simulink model "Solar_App"  (R2020a)
settings: Solver=VariableStepAuto  StartTime=0.0  StopTime=10.0  RelTol=1e-3
libraries: ee_lib x81, powerlib x29, fl_lib x4, nesl_utility x3, powerlib_extras x1
settings Model: Creator=momit  LastModifiedBy=royde
settings DataIOCC: ReturnWorkspaceOutputs=off
settings DebuggingCC: ArithmeticOperatorsInVariantConditions=warning
settings SFSimCC: SimUseLocalCustomCode=off  CustomCodeUndefinedFunction=UseInterfaceOnly
settings RTWCC: RTWUseLocalCustomCode=off

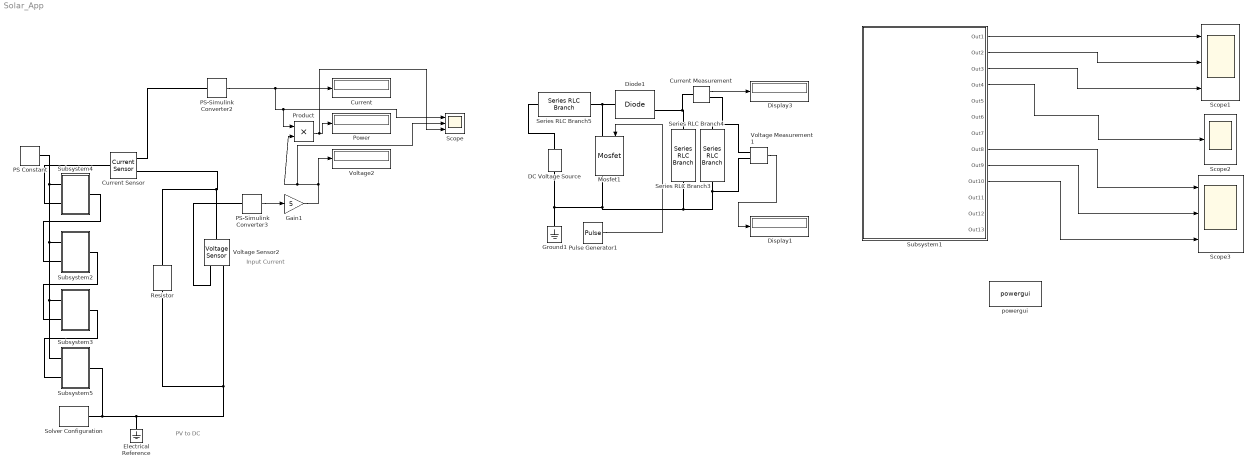
== system Solar_App ==
  note: Input Current
  note: PV to DC
  Current : Display
  Current Measurement : powerlib/Measurements/Current Measurement  PhasorSimulation=off  OutputType=Complex  PSBequivalent=0
  Current Sensor : fl_lib/Electrical/Electrical Sensors/Current Sensor
  DC Voltage Source : powerlib/Electrical Sources/DC Voltage Source  Amplitude=29.36  Measurements=None
  Diode1 : powerlib/Power Electronics/Diode  Ron=0.001  Lon=0  Vf=0.8  IC=0  UseSnubber=0  Rs=500  Cs=250e-9  Measurements=on
  Display1 : Display
  Display3 : Display
  Electrical Reference : fl_lib/Electrical/Electrical Elements/Electrical Reference
  Gain1 : Gain  Gain=5
  Ground1 : powerlib/Elements/Ground  LConnTagsString=a
  Mosfet1 : powerlib/Power Electronics/Mosfet  Ron=0.001  Lon=0  Rd=0.001  Vfd=0  IC=0  Rs=1e5  Cs=inf  Measurements=on
  PS Constant : fl_lib/Physical Signals/Sources/PS Constant  constant=1000
  PS-Simulink Converter2 : nesl_utility/PS-Simulink Converter  PhysicalDomain=network_engine_domain  SubClassName=ps_output  LeftPortType=input  RightPortType=output  PseudoPeriodic=off  Frequencies=[]  Unit=1  AffineConversion=off
  PS-Simulink Converter3 : nesl_utility/PS-Simulink Converter  PhysicalDomain=network_engine_domain  SubClassName=ps_output  LeftPortType=input  RightPortType=output  PseudoPeriodic=off  Frequencies=[]  Unit=1  AffineConversion=off
  Power : Display
  Product : Product
  Pulse Generator1 : DiscretePulseGenerator  PulseType=Time based  Period=1/25000  PulseWidth=75
  Resistor : ee_lib/Passive/Resistor  R=1 Ohm  R_tol=5  enable_R_tol=0  tol_distribution=1  nSigma=4  enable_operating_limits=0  operating_limit_action=2  max_working_voltage=100 V  power_rating=1 W  enable_faults=0  fault_action=1  R_faulted=inf Ohm  enable_temporal_fault=0  t_fault=1 s  enable_behavioral_fault=0  max_permissible_current=1 A  t_fail_on_current=1 s  noise_mode=0  sample_time=1e-3 s  repeatability=1  auto_seed=1196140742  user_seed=0  Tdevice=25 degC  alpha=3.93e-3 1/K  Tmeas=25 degC  thermal_mass=100 J/K  power_derating_T1=70 degC  power_derating_T2=155 degC  operating_temperature_range_vec=[-50, 150] degC  temperature_specify=off  temperature_priority=High  temperature=298.15 K  temperature_nominal_specify=off  temperature_nominal_unit=K  temperature_nominal_value=1
  Scope : Scope  NumInputPorts=3
  Scope1 : Scope  NumInputPorts=3
  Scope2 : Scope
  Scope3 : Scope  NumInputPorts=3
  Series RLC Branch3 : powerlib/Elements/Series RLC Branch  LConnTagsString=__new0  RConnTagsString=__new0  BranchType=C  Resistance=1  Inductance=1e-3  SetiL0=off  InitialCurrent=0  Capacitance=1e-6  Setx0=off  InitialVoltage=0  Measurements=None
  Series RLC Branch4 : powerlib/Elements/Series RLC Branch  LConnTagsString=__new0  RConnTagsString=__new0  BranchType=R  Resistance=100  Inductance=1e-3  SetiL0=off  InitialCurrent=0  Capacitance=1e-6  Setx0=off  InitialVoltage=0  Measurements=None
  Series RLC Branch5 : powerlib/Elements/Series RLC Branch  LConnTagsString=__new0  RConnTagsString=__new0  BranchType=L  Resistance=1  Inductance=1e-3  SetiL0=off  InitialCurrent=0  Capacitance=1e-6  Setx0=off  InitialVoltage=0  Measurements=None
  Solver Configuration : nesl_utility/Solver Configuration  PhysicalDomain=network_engine_domain  SubClassName=solver  LeftPortType=input  RightPortType=generic  Tones=[]  Harmonics=[]  SimulateNoise=off  Profile=off  UseLocalSampling=off  EnableSwitchedLinearOptims=on  FrequencyDomain=off  UseCCode=off  RelTol=0.001  AbsTol=1e-06  MinStep=1e-09  ToWorkspace=off  RevertToSquareIcSolve=off  NumHomotopyIterations=100  PhasorMode=off  PhasorModeNumHarmonics=1  DoDC=off  ResidualTolerance=1e-09  UseLocalSolver=off  LocalSolverChoice=NE_BACKWARD_EULER_ADVANCER  LocalSolverSampleTime=0.001  DoFixedCost=off  MaxNonlinIter=3  MaxModeIter=2  LinearAlgebra=Sparse  EquationFormulation=NE_TIME_EF  DelaysMemoryBudget=1024  AutomaticFiltering=on  FilteringTimeConstant=0.001  PartitionStorageMethod=AS_NEEDED  PartitionMemoryBudget=1024  PartitionMethod=FAST
  Subsystem1 : Subsystem
  Subsystem2 : Subsystem
  Subsystem3 : Subsystem
  Subsystem4 : Subsystem
  Subsystem5 : Subsystem
  Voltage Measurement1 : powerlib/Measurements/Voltage Measurement  PhasorSimulation=off  OutputType=Complex  PSBequivalent=0
  Voltage Sensor2 : fl_lib/Electrical/Electrical Sensors/Voltage Sensor
  Voltage2 : Display
  powergui : powerlib/powergui  Priority=1  SimulationMode=Continuous  SampleTime=50e-6  frequency=60  Iterations=50  frequencyindice=0  Pbase=100e6  ErrMax=1e-4  UnitsV=kV  UnitsW=MW  buscounter=0  FunctionMessages=off  echomessages=off  EnableUseOfTLC=off  CurrentSourceSwitches=off  DisableSnubberDevices=off  DisableRonSwitches=off  DisableVfSwitches=off  DisplayEquations=off  AutomaticDiscreteSolvers=off  SolverType=Tustin/Backward Euler (TBE)  Interpol=off  ExternalGateDelay=off  methode=off  Ts=100  x0status=blocks  SPID=on  SwTol=0  HookPort=off  NonlinearTolerance=1e-4  nMaxIteration=100  ContinueOnMaxIteration=off  RestoreLinks=warning  ResistiveCurrentMeasurement=off  Frange=[0:2:500]  Ylog=off  Xlog=on  ShowGrid=off  save=off  variable=ZData  structure=0  ZoomFFT=off  StartTime=0.0  cycles=1  DisplayStyle=1  fundamental=60  FreqAxis=off  MaxFrequency=1000  frequencyindicesteady=1  RmsSteady=1  display=off
  wires:
  Voltage Measurement1/1 -> Display1/1
  Pulse Generator1/1 -> Mosfet1/1
  Subsystem1/1(Out1) -> Scope1/1
  Subsystem1/2(Out2) -> Scope1/2
  Subsystem1/3(Out3) -> Scope1/3
  Subsystem1/4(Out4) -> Scope2/1
  Subsystem1/8(Out8) -> Scope3/1
  Subsystem1/9(Out9) -> Scope3/2
  Subsystem1/10(Out10) -> Scope3/3
  Current Measurement/1 -> Display3/1
  Gain1/1 -> Scope/2, Product/2, Voltage2/1
  PS-Simulink Converter2/1 -> Product/1, Scope/1, Current/1
  Product/1 -> Scope/3, Power/1
  PS-Simulink Converter3/1 -> Gain1/1
  connections:
  DC Voltage Source/LConn1 -- Ground1/LConn1 -- Series RLC Branch4/RConn1 -- Voltage Measurement1/LConn2 -- Series RLC Branch3/RConn1 -- Mosfet1/RConn1
  Series RLC Branch3/LConn1 -- Current Measurement/LConn1 -- Diode1/RConn1
  Diode1/LConn1 -- Series RLC Branch5/RConn1 -- Mosfet1/LConn1
  DC Voltage Source/RConn1 -- Series RLC Branch5/LConn1
  Voltage Measurement1/LConn1 -- Current Measurement/RConn1 -- Series RLC Branch4/LConn1
  Voltage Sensor2/LConn1 -- Resistor/LConn1 -- Current Sensor/RConn2
  Voltage Sensor2/RConn2 -- Resistor/RConn1 -- Electrical Reference/LConn1 -- Solver Configuration/RConn1 -- Subsystem5/RConn1
  Subsystem3/LConn1 -- PS Constant/RConn1 -- Subsystem4/LConn1 -- Subsystem2/LConn1 -- Subsystem5/LConn1
  Subsystem2/LConn2 -- Subsystem4/RConn1
  Voltage Sensor2/RConn1 -- PS-Simulink Converter3/LConn1
  Subsystem4/LConn2 -- Current Sensor/LConn1
  Subsystem3/LConn2 -- Subsystem2/RConn1
  Current Sensor/RConn1 -- PS-Simulink Converter2/LConn1
  Subsystem5/LConn2 -- Subsystem3/RConn1

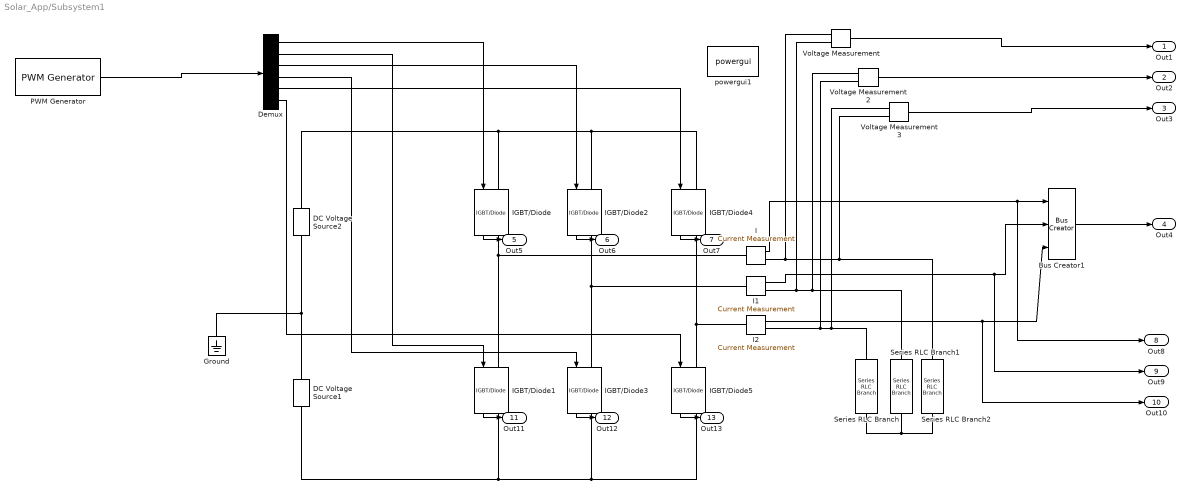
== system Solar_App/Subsystem1 ==
  Bus Creator1 : BusCreator  Inputs=3
  DC Voltage Source1 : powerlib/Electrical Sources/DC Voltage Source  Amplitude=215.3  Measurements=None
  DC Voltage Source2 : powerlib/Electrical Sources/DC Voltage Source  Amplitude=215.3  Measurements=None
  Demux : Demux  Outputs=6
  Ground : powerlib/Elements/Ground  LConnTagsString=a
  I : powerlib/Measurements/Current Measurement  PhasorSimulation=off  OutputType=Complex  PSBequivalent=0
  I1 : powerlib/Measurements/Current Measurement  PhasorSimulation=off  OutputType=Complex  PSBequivalent=0
  I2 : powerlib/Measurements/Current Measurement  PhasorSimulation=off  OutputType=Complex  PSBequivalent=0
  IGBT/Diode{,1..5} (6 alike) : powerlib/Power Electronics/IGBT//Diode  Ron=1e-3  Rs=1e5  Cs=inf  Measurements=on
  PWM Generator : powerlib_extras/Control  Blocks/PWM Generator  GeneratorMode="3-arm  bridge (6 pulses)"  Fc=10000  Internal=on  mIndex=0.8  Freq=50  Phase=0
      settings: SourceProductBaseCode=PS
  Series RLC Branch : powerlib/Elements/Series RLC Branch  LConnTagsString=__new0  RConnTagsString=__new0  BranchType=RL  Resistance=1.5  Inductance=1e-3  SetiL0=off  InitialCurrent=0  Capacitance=1e-6  Setx0=off  InitialVoltage=0  Measurements=None
  Series RLC Branch1 : powerlib/Elements/Series RLC Branch  LConnTagsString=__new0  RConnTagsString=__new0  BranchType=RL  Resistance=1.5  Inductance=1e-3  SetiL0=off  InitialCurrent=0  Capacitance=1e-6  Setx0=off  InitialVoltage=0  Measurements=None
  Series RLC Branch2 : powerlib/Elements/Series RLC Branch  LConnTagsString=__new0  RConnTagsString=__new0  BranchType=RL  Resistance=1.5  Inductance=1e-3  SetiL0=off  InitialCurrent=0  Capacitance=1e-6  Setx0=off  InitialVoltage=0  Measurements=None
  Voltage Measurement : powerlib/Measurements/Voltage Measurement  PhasorSimulation=off  OutputType=Complex  PSBequivalent=0
  Voltage Measurement2 : powerlib/Measurements/Voltage Measurement  PhasorSimulation=off  OutputType=Complex  PSBequivalent=0
  Voltage Measurement3 : powerlib/Measurements/Voltage Measurement  PhasorSimulation=off  OutputType=Complex  PSBequivalent=0
  powergui1 : powerlib/powergui  Priority=1  SimulationMode=Continuous  SampleTime=50e-6  frequency=60  Iterations=50  frequencyindice=0  Pbase=100e6  ErrMax=1e-4  UnitsV=kV  UnitsW=MW  buscounter=0  FunctionMessages=off  echomessages=off  EnableUseOfTLC=off  CurrentSourceSwitches=on  DisableSnubberDevices=off  DisableRonSwitches=off  DisableVfSwitches=off  DisplayEquations=off  AutomaticDiscreteSolvers=off  SolverType=Tustin  Interpol=off  ExternalGateDelay=off  methode=off  Ts=100  x0status=blocks  SPID=off  SwTol=0  HookPort=off  NonlinearTolerance=1e-4  nMaxIteration=100  ContinueOnMaxIteration=off  RestoreLinks=warning  ResistiveCurrentMeasurement=off  Frange=[0:2:500]  Ylog=off  Xlog=on  ShowGrid=off  save=off  variable=ZData  structure=ScopeData2  ZoomFFT=off  StartTime=0.0  cycles=1  DisplayStyle=1  fundamental=50  FreqAxis=off  MaxFrequency=1000  frequencyindicesteady=1  RmsSteady=1  display=off
  Out1 : Outport  VectorParamsAs1DForOutWhenUnconnected=off
  Out2 : Outport  Port=2  VectorParamsAs1DForOutWhenUnconnected=off
  Out3 : Outport  Port=3  VectorParamsAs1DForOutWhenUnconnected=off
  Out4 : Outport  Port=4  VectorParamsAs1DForOutWhenUnconnected=off
  Out5 : Outport  Port=5  VectorParamsAs1DForOutWhenUnconnected=off
  Out6 : Outport  Port=6  VectorParamsAs1DForOutWhenUnconnected=off
  Out7 : Outport  Port=7  VectorParamsAs1DForOutWhenUnconnected=off
  Out8 : Outport  Port=8  VectorParamsAs1DForOutWhenUnconnected=off
  Out9 : Outport  Port=9  VectorParamsAs1DForOutWhenUnconnected=off
  Out10 : Outport  Port=10  VectorParamsAs1DForOutWhenUnconnected=off
  Out11 : Outport  Port=11  VectorParamsAs1DForOutWhenUnconnected=off
  Out12 : Outport  Port=12  VectorParamsAs1DForOutWhenUnconnected=off
  Out13 : Outport  Port=13  VectorParamsAs1DForOutWhenUnconnected=off
  wires:
  IGBT/Diode/1 -> Out5/1
  I1/1 -> Out9/1, Bus Creator1/2
  I2/1 -> Out10/1, Bus Creator1/3
  Demux/2 -> IGBT/Diode1/1
  Demux/5 -> IGBT/Diode4/1
  PWM Generator/1 -> Demux/1
  IGBT/Diode4/1 -> Out7/1
  I/1 -> Out8/1, Bus Creator1/1
  Bus Creator1/1 -> Out4/1
  IGBT/Diode5/1 -> Out13/1
  Demux/1 -> IGBT/Diode/1
  Demux/4 -> IGBT/Diode3/1
  Demux/6 -> IGBT/Diode5/1
  Demux/3 -> IGBT/Diode2/1
  Voltage Measurement/1 -> Out1/1
  IGBT/Diode2/1 -> Out6/1
  Voltage Measurement2/1 -> Out2/1
  IGBT/Diode1/1 -> Out11/1
  Voltage Measurement3/1 -> Out3/1
  IGBT/Diode3/1 -> Out12/1
  connections:
  IGBT/Diode2/LConn1 -- IGBT/Diode/LConn1 -- DC Voltage Source2/RConn1 -- IGBT/Diode4/LConn1
  I/LConn1 -- IGBT/Diode/RConn1 -- IGBT/Diode1/LConn1
  Ground/LConn1 -- DC Voltage Source2/LConn1 -- DC Voltage Source1/RConn1
  Voltage Measurement3/LConn1 -- Series RLC Branch/LConn1 -- I2/RConn1 -- Voltage Measurement2/LConn2
  I1/LConn1 -- IGBT/Diode3/LConn1 -- IGBT/Diode2/RConn1
  Voltage Measurement/LConn2 -- Series RLC Branch1/LConn1 -- Voltage Measurement2/LConn1 -- I1/RConn1
  IGBT/Diode5/RConn1 -- IGBT/Diode1/RConn1 -- DC Voltage Source1/LConn1 -- IGBT/Diode3/RConn1
  Series RLC Branch1/RConn1 -- Series RLC Branch/RConn1 -- Series RLC Branch2/RConn1
  Voltage Measurement3/LConn2 -- I/RConn1 -- Voltage Measurement/LConn1 -- Series RLC Branch2/LConn1
  I2/LConn1 -- IGBT/Diode4/RConn1 -- IGBT/Diode5/LConn1

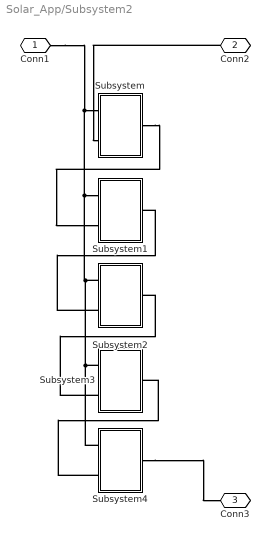
== system Solar_App/Subsystem2 ==
  Subsystem : Subsystem
  Subsystem1 : Subsystem
  Subsystem2 : Subsystem
  Subsystem3 : Subsystem
  Subsystem4 : Subsystem
  Conn1 : PMIOPort  Side=Left
  Conn2 : PMIOPort  Port=2  Side=Left
  Conn3 : PMIOPort  Port=3  Side=Right
  connections:
  Subsystem4/RConn1 -- Conn3/RConn1
  Subsystem4/LConn2 -- Subsystem3/RConn1
  Subsystem3/LConn2 -- Subsystem2/RConn1
  Conn2/RConn1 -- Subsystem/LConn2
  Subsystem/RConn1 -- Subsystem1/LConn2
  Subsystem2/LConn2 -- Subsystem1/RConn1
  Subsystem4/LConn1 -- Conn1/RConn1 -- Subsystem/LConn1 -- Subsystem1/LConn1 -- Subsystem2/LConn1 -- Subsystem3/LConn1

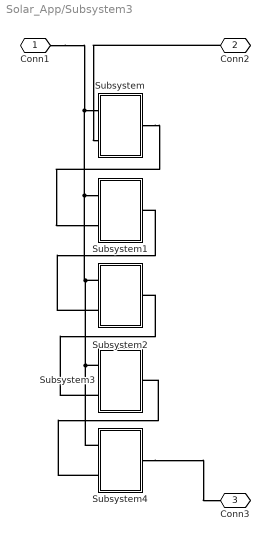
== system Solar_App/Subsystem3 ==
  Subsystem : Subsystem
  Subsystem1 : Subsystem
  Subsystem2 : Subsystem
  Subsystem3 : Subsystem
  Subsystem4 : Subsystem
  Conn1 : PMIOPort  Side=Left
  Conn2 : PMIOPort  Port=2  Side=Left
  Conn3 : PMIOPort  Port=3  Side=Right
  connections:
  Subsystem3/LConn1 -- Subsystem2/LConn1 -- Subsystem1/LConn1 -- Subsystem/LConn1 -- Conn1/RConn1 -- Subsystem4/LConn1
  Subsystem2/LConn2 -- Subsystem1/RConn1
  Subsystem/RConn1 -- Subsystem1/LConn2
  Conn2/RConn1 -- Subsystem/LConn2
  Subsystem3/LConn2 -- Subsystem2/RConn1
  Subsystem4/LConn2 -- Subsystem3/RConn1
  Subsystem4/RConn1 -- Conn3/RConn1

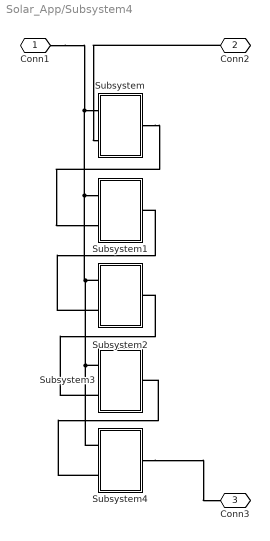
== system Solar_App/Subsystem4 ==
  Subsystem : Subsystem
  Subsystem1 : Subsystem
  Subsystem2 : Subsystem
  Subsystem3 : Subsystem
  Subsystem4 : Subsystem
  Conn1 : PMIOPort  Side=Left
  Conn2 : PMIOPort  Port=2  Side=Left
  Conn3 : PMIOPort  Port=3  Side=Right
  connections:
  Conn1/RConn1 -- Subsystem/LConn1 -- Subsystem2/LConn1 -- Subsystem4/LConn1 -- Subsystem3/LConn1 -- Subsystem1/LConn1
  Subsystem2/LConn2 -- Subsystem1/RConn1
  Subsystem/RConn1 -- Subsystem1/LConn2
  Conn2/RConn1 -- Subsystem/LConn2
  Subsystem3/LConn2 -- Subsystem2/RConn1
  Subsystem4/LConn2 -- Subsystem3/RConn1
  Subsystem4/RConn1 -- Conn3/RConn1

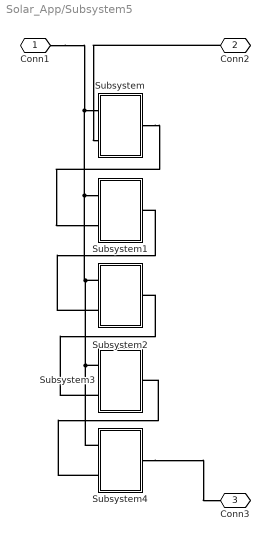
== system Solar_App/Subsystem5 ==
  Subsystem : Subsystem
  Subsystem1 : Subsystem
  Subsystem2 : Subsystem
  Subsystem3 : Subsystem
  Subsystem4 : Subsystem
  Conn1 : PMIOPort  Side=Left
  Conn2 : PMIOPort  Port=2  Side=Left
  Conn3 : PMIOPort  Port=3  Side=Right
  connections:
  Subsystem4/RConn1 -- Conn3/RConn1
  Subsystem4/LConn2 -- Subsystem3/RConn1
  Subsystem3/LConn2 -- Subsystem2/RConn1
  Conn2/RConn1 -- Subsystem/LConn2
  Subsystem/RConn1 -- Subsystem1/LConn2
  Subsystem2/LConn2 -- Subsystem1/RConn1
  Subsystem4/LConn1 -- Conn1/RConn1 -- Subsystem/LConn1 -- Subsystem1/LConn1 -- Subsystem2/LConn1 -- Subsystem3/LConn1

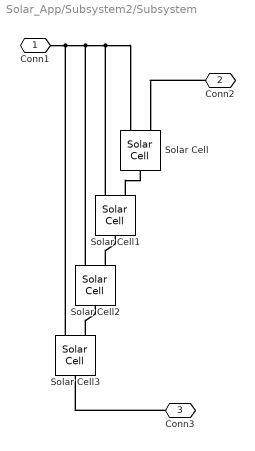
== system Solar_App/Subsystem2/Subsystem ==
  Solar Cell{,1..3} (4 alike) : ee_lib/Sources/Solar Cell  prm=1  Isc=7.34 A  Voc=0.6 V  Is=1e-6 A  Is2=0 A  Iph=7.34 A  Ir0=1000 W/m^2  ec=1.5  N2=2  Rs=0 Ohm  Rp=inf Ohm  N_series=1  TIPH1=0 1/K  EG=1.11 eV  TXIS1=3  TXIS2=3  TRS1=0  TRP1=0  Tmeas=25 degC  TFIXED=25 degC  thermal_mass=100 J/K  initial_temperature=25 degC
      settings: SourceProductBaseCode=PS
  Conn1 : PMIOPort  Side=Left
  Conn2 : PMIOPort  Port=2  Side=Left
  Conn3 : PMIOPort  Port=3  Side=Right
  connections:
  Conn3/RConn1 -- Solar Cell3/RConn1
  Solar Cell3/LConn2 -- Solar Cell2/RConn1
  Solar Cell2/LConn2 -- Solar Cell1/RConn1
  Solar Cell1/LConn2 -- Solar Cell/RConn1
  Conn2/RConn1 -- Solar Cell/LConn2
  Solar Cell3/LConn1 -- Conn1/RConn1 -- Solar Cell2/LConn1 -- Solar Cell1/LConn1 -- Solar Cell/LConn1

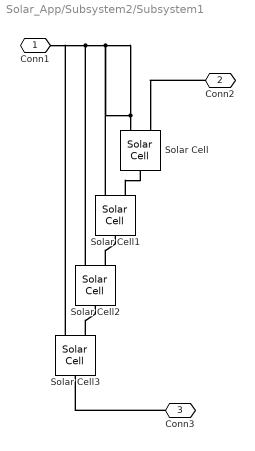
== system Solar_App/Subsystem2/Subsystem1 ==
  Solar Cell{,1..3} (4 alike) : ee_lib/Sources/Solar Cell  prm=1  Isc=7.34 A  Voc=0.6 V  Is=1e-6 A  Is2=0 A  Iph=7.34 A  Ir0=1000 W/m^2  ec=1.5  N2=2  Rs=0 Ohm  Rp=inf Ohm  N_series=1  TIPH1=0 1/K  EG=1.11 eV  TXIS1=3  TXIS2=3  TRS1=0  TRP1=0  Tmeas=25 degC  TFIXED=25 degC  thermal_mass=100 J/K  initial_temperature=25 degC
      settings: SourceProductBaseCode=PS
  Conn1 : PMIOPort  Side=Left
  Conn2 : PMIOPort  Port=2  Side=Left
  Conn3 : PMIOPort  Port=3  Side=Right
  connections:
  Solar Cell/LConn1 -- Solar Cell1/LConn1 -- Solar Cell2/LConn1 -- Conn1/RConn1 -- Solar Cell3/LConn1
  Conn2/RConn1 -- Solar Cell/LConn2
  Solar Cell1/LConn2 -- Solar Cell/RConn1
  Solar Cell2/LConn2 -- Solar Cell1/RConn1
  Solar Cell3/LConn2 -- Solar Cell2/RConn1
  Conn3/RConn1 -- Solar Cell3/RConn1

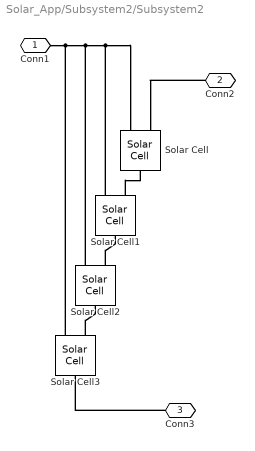
== system Solar_App/Subsystem2/Subsystem2 ==
  Solar Cell{,1..3} (4 alike) : ee_lib/Sources/Solar Cell  prm=1  Isc=7.34 A  Voc=0.6 V  Is=1e-6 A  Is2=0 A  Iph=7.34 A  Ir0=1000 W/m^2  ec=1.5  N2=2  Rs=0 Ohm  Rp=inf Ohm  N_series=1  TIPH1=0 1/K  EG=1.11 eV  TXIS1=3  TXIS2=3  TRS1=0  TRP1=0  Tmeas=25 degC  TFIXED=25 degC  thermal_mass=100 J/K  initial_temperature=25 degC
      settings: SourceProductBaseCode=PS
  Conn1 : PMIOPort  Side=Left
  Conn2 : PMIOPort  Port=2  Side=Left
  Conn3 : PMIOPort  Port=3  Side=Right
  connections:
  Conn3/RConn1 -- Solar Cell3/RConn1
  Solar Cell3/LConn2 -- Solar Cell2/RConn1
  Solar Cell2/LConn2 -- Solar Cell1/RConn1
  Solar Cell1/LConn2 -- Solar Cell/RConn1
  Conn2/RConn1 -- Solar Cell/LConn2
  Solar Cell3/LConn1 -- Conn1/RConn1 -- Solar Cell2/LConn1 -- Solar Cell1/LConn1 -- Solar Cell/LConn1

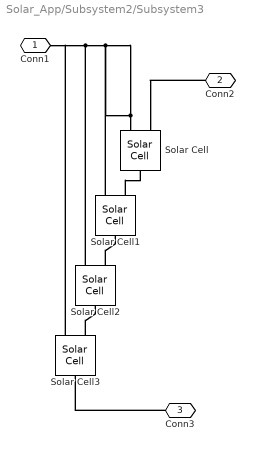
== system Solar_App/Subsystem2/Subsystem3 ==
  Solar Cell{,1..3} (4 alike) : ee_lib/Sources/Solar Cell  prm=1  Isc=7.34 A  Voc=0.6 V  Is=1e-6 A  Is2=0 A  Iph=7.34 A  Ir0=1000 W/m^2  ec=1.5  N2=2  Rs=0 Ohm  Rp=inf Ohm  N_series=1  TIPH1=0 1/K  EG=1.11 eV  TXIS1=3  TXIS2=3  TRS1=0  TRP1=0  Tmeas=25 degC  TFIXED=25 degC  thermal_mass=100 J/K  initial_temperature=25 degC
      settings: SourceProductBaseCode=PS
  Conn1 : PMIOPort  Side=Left
  Conn2 : PMIOPort  Port=2  Side=Left
  Conn3 : PMIOPort  Port=3  Side=Right
  connections:
  Solar Cell/LConn1 -- Solar Cell1/LConn1 -- Solar Cell2/LConn1 -- Conn1/RConn1 -- Solar Cell3/LConn1
  Conn2/RConn1 -- Solar Cell/LConn2
  Solar Cell1/LConn2 -- Solar Cell/RConn1
  Solar Cell2/LConn2 -- Solar Cell1/RConn1
  Solar Cell3/LConn2 -- Solar Cell2/RConn1
  Conn3/RConn1 -- Solar Cell3/RConn1

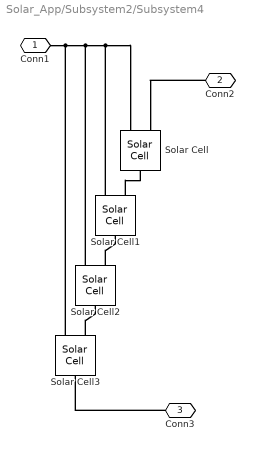
== system Solar_App/Subsystem2/Subsystem4 ==
  Solar Cell{,1..3} (4 alike) : ee_lib/Sources/Solar Cell  prm=1  Isc=7.34 A  Voc=0.6 V  Is=1e-6 A  Is2=0 A  Iph=7.34 A  Ir0=1000 W/m^2  ec=1.5  N2=2  Rs=0 Ohm  Rp=inf Ohm  N_series=1  TIPH1=0 1/K  EG=1.11 eV  TXIS1=3  TXIS2=3  TRS1=0  TRP1=0  Tmeas=25 degC  TFIXED=25 degC  thermal_mass=100 J/K  initial_temperature=25 degC
      settings: SourceProductBaseCode=PS
  Conn1 : PMIOPort  Side=Left
  Conn2 : PMIOPort  Port=2  Side=Left
  Conn3 : PMIOPort  Port=3  Side=Right
  connections:
  Conn3/RConn1 -- Solar Cell3/RConn1
  Solar Cell3/LConn2 -- Solar Cell2/RConn1
  Solar Cell2/LConn2 -- Solar Cell1/RConn1
  Solar Cell1/LConn2 -- Solar Cell/RConn1
  Conn2/RConn1 -- Solar Cell/LConn2
  Solar Cell3/LConn1 -- Conn1/RConn1 -- Solar Cell2/LConn1 -- Solar Cell1/LConn1 -- Solar Cell/LConn1

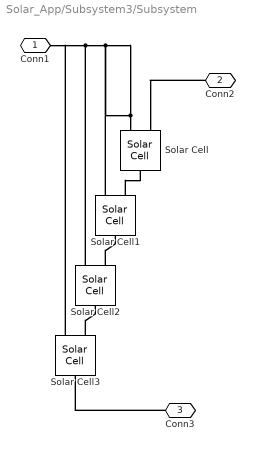
== system Solar_App/Subsystem3/Subsystem ==
  Solar Cell{,1..3} (4 alike) : ee_lib/Sources/Solar Cell  prm=1  Isc=7.34 A  Voc=0.6 V  Is=1e-6 A  Is2=0 A  Iph=7.34 A  Ir0=1000 W/m^2  ec=1.5  N2=2  Rs=0 Ohm  Rp=inf Ohm  N_series=1  TIPH1=0 1/K  EG=1.11 eV  TXIS1=3  TXIS2=3  TRS1=0  TRP1=0  Tmeas=25 degC  TFIXED=25 degC  thermal_mass=100 J/K  initial_temperature=25 degC
      settings: SourceProductBaseCode=PS
  Conn1 : PMIOPort  Side=Left
  Conn2 : PMIOPort  Port=2  Side=Left
  Conn3 : PMIOPort  Port=3  Side=Right
  connections:
  Solar Cell/LConn1 -- Solar Cell1/LConn1 -- Solar Cell2/LConn1 -- Conn1/RConn1 -- Solar Cell3/LConn1
  Conn2/RConn1 -- Solar Cell/LConn2
  Solar Cell1/LConn2 -- Solar Cell/RConn1
  Solar Cell2/LConn2 -- Solar Cell1/RConn1
  Solar Cell3/LConn2 -- Solar Cell2/RConn1
  Conn3/RConn1 -- Solar Cell3/RConn1

== system Solar_App/Subsystem3/Subsystem1 ==
  Solar Cell{,1..3} (4 alike) : ee_lib/Sources/Solar Cell  prm=1  Isc=7.34 A  Voc=0.6 V  Is=1e-6 A  Is2=0 A  Iph=7.34 A  Ir0=1000 W/m^2  ec=1.5  N2=2  Rs=0 Ohm  Rp=inf Ohm  N_series=1  TIPH1=0 1/K  EG=1.11 eV  TXIS1=3  TXIS2=3  TRS1=0  TRP1=0  Tmeas=25 degC  TFIXED=25 degC  thermal_mass=100 J/K  initial_temperature=25 degC
      settings: SourceProductBaseCode=PS
  Conn1 : PMIOPort  Side=Left
  Conn2 : PMIOPort  Port=2  Side=Left
  Conn3 : PMIOPort  Port=3  Side=Right
  connections:
  Conn3/RConn1 -- Solar Cell3/RConn1
  Solar Cell3/LConn2 -- Solar Cell2/RConn1
  Solar Cell2/LConn2 -- Solar Cell1/RConn1
  Solar Cell1/LConn2 -- Solar Cell/RConn1
  Conn2/RConn1 -- Solar Cell/LConn2
  Solar Cell3/LConn1 -- Conn1/RConn1 -- Solar Cell2/LConn1 -- Solar Cell1/LConn1 -- Solar Cell/LConn1

== system Solar_App/Subsystem3/Subsystem2 ==
  Solar Cell{,1..3} (4 alike) : ee_lib/Sources/Solar Cell  prm=1  Isc=7.34 A  Voc=0.6 V  Is=1e-6 A  Is2=0 A  Iph=7.34 A  Ir0=1000 W/m^2  ec=1.5  N2=2  Rs=0 Ohm  Rp=inf Ohm  N_series=1  TIPH1=0 1/K  EG=1.11 eV  TXIS1=3  TXIS2=3  TRS1=0  TRP1=0  Tmeas=25 degC  TFIXED=25 degC  thermal_mass=100 J/K  initial_temperature=25 degC
      settings: SourceProductBaseCode=PS
  Conn1 : PMIOPort  Side=Left
  Conn2 : PMIOPort  Port=2  Side=Left
  Conn3 : PMIOPort  Port=3  Side=Right
  connections:
  Solar Cell/LConn1 -- Solar Cell1/LConn1 -- Solar Cell2/LConn1 -- Conn1/RConn1 -- Solar Cell3/LConn1
  Conn2/RConn1 -- Solar Cell/LConn2
  Solar Cell1/LConn2 -- Solar Cell/RConn1
  Solar Cell2/LConn2 -- Solar Cell1/RConn1
  Solar Cell3/LConn2 -- Solar Cell2/RConn1
  Conn3/RConn1 -- Solar Cell3/RConn1

== system Solar_App/Subsystem3/Subsystem3 ==
  Solar Cell{,1..3} (4 alike) : ee_lib/Sources/Solar Cell  prm=1  Isc=7.34 A  Voc=0.6 V  Is=1e-6 A  Is2=0 A  Iph=7.34 A  Ir0=1000 W/m^2  ec=1.5  N2=2  Rs=0 Ohm  Rp=inf Ohm  N_series=1  TIPH1=0 1/K  EG=1.11 eV  TXIS1=3  TXIS2=3  TRS1=0  TRP1=0  Tmeas=25 degC  TFIXED=25 degC  thermal_mass=100 J/K  initial_temperature=25 degC
      settings: SourceProductBaseCode=PS
  Conn1 : PMIOPort  Side=Left
  Conn2 : PMIOPort  Port=2  Side=Left
  Conn3 : PMIOPort  Port=3  Side=Right
  connections:
  Conn3/RConn1 -- Solar Cell3/RConn1
  Solar Cell3/LConn2 -- Solar Cell2/RConn1
  Solar Cell2/LConn2 -- Solar Cell1/RConn1
  Solar Cell1/LConn2 -- Solar Cell/RConn1
  Conn2/RConn1 -- Solar Cell/LConn2
  Solar Cell3/LConn1 -- Conn1/RConn1 -- Solar Cell2/LConn1 -- Solar Cell1/LConn1 -- Solar Cell/LConn1

== system Solar_App/Subsystem3/Subsystem4 ==
  Solar Cell{,1..3} (4 alike) : ee_lib/Sources/Solar Cell  prm=1  Isc=7.34 A  Voc=0.6 V  Is=1e-6 A  Is2=0 A  Iph=7.34 A  Ir0=1000 W/m^2  ec=1.5  N2=2  Rs=0 Ohm  Rp=inf Ohm  N_series=1  TIPH1=0 1/K  EG=1.11 eV  TXIS1=3  TXIS2=3  TRS1=0  TRP1=0  Tmeas=25 degC  TFIXED=25 degC  thermal_mass=100 J/K  initial_temperature=25 degC
      settings: SourceProductBaseCode=PS
  Conn1 : PMIOPort  Side=Left
  Conn2 : PMIOPort  Port=2  Side=Left
  Conn3 : PMIOPort  Port=3  Side=Right
  connections:
  Solar Cell/LConn1 -- Solar Cell1/LConn1 -- Solar Cell2/LConn1 -- Conn1/RConn1 -- Solar Cell3/LConn1
  Conn2/RConn1 -- Solar Cell/LConn2
  Solar Cell1/LConn2 -- Solar Cell/RConn1
  Solar Cell2/LConn2 -- Solar Cell1/RConn1
  Solar Cell3/LConn2 -- Solar Cell2/RConn1
  Conn3/RConn1 -- Solar Cell3/RConn1

== system Solar_App/Subsystem4/Subsystem ==
  Solar Cell{,1..3} (4 alike) : ee_lib/Sources/Solar Cell  prm=1  Isc=7.34 A  Voc=0.6 V  Is=1e-6 A  Is2=0 A  Iph=7.34 A  Ir0=1000 W/m^2  ec=1.5  N2=2  Rs=0 Ohm  Rp=inf Ohm  N_series=1  TIPH1=0 1/K  EG=1.11 eV  TXIS1=3  TXIS2=3  TRS1=0  TRP1=0  Tmeas=25 degC  TFIXED=25 degC  thermal_mass=100 J/K  initial_temperature=25 degC
      settings: SourceProductBaseCode=PS
  Conn1 : PMIOPort  Side=Left
  Conn2 : PMIOPort  Port=2  Side=Left
  Conn3 : PMIOPort  Port=3  Side=Right
  connections:
  Solar Cell/LConn1 -- Solar Cell3/LConn1 -- Conn1/RConn1 -- Solar Cell2/LConn1 -- Solar Cell1/LConn1
  Conn2/RConn1 -- Solar Cell/LConn2
  Solar Cell1/LConn2 -- Solar Cell/RConn1
  Solar Cell2/LConn2 -- Solar Cell1/RConn1
  Solar Cell3/LConn2 -- Solar Cell2/RConn1
  Conn3/RConn1 -- Solar Cell3/RConn1

== system Solar_App/Subsystem4/Subsystem1 ==
  Solar Cell{,1..3} (4 alike) : ee_lib/Sources/Solar Cell  prm=1  Isc=7.34 A  Voc=0.6 V  Is=1e-6 A  Is2=0 A  Iph=7.34 A  Ir0=1000 W/m^2  ec=1.5  N2=2  Rs=0 Ohm  Rp=inf Ohm  N_series=1  TIPH1=0 1/K  EG=1.11 eV  TXIS1=3  TXIS2=3  TRS1=0  TRP1=0  Tmeas=25 degC  TFIXED=25 degC  thermal_mass=100 J/K  initial_temperature=25 degC
      settings: SourceProductBaseCode=PS
  Conn1 : PMIOPort  Side=Left
  Conn2 : PMIOPort  Port=2  Side=Left
  Conn3 : PMIOPort  Port=3  Side=Right
  connections:
  Conn3/RConn1 -- Solar Cell3/RConn1
  Solar Cell3/LConn2 -- Solar Cell2/RConn1
  Solar Cell2/LConn2 -- Solar Cell1/RConn1
  Solar Cell1/LConn2 -- Solar Cell/RConn1
  Conn2/RConn1 -- Solar Cell/LConn2
  Solar Cell3/LConn1 -- Conn1/RConn1 -- Solar Cell2/LConn1 -- Solar Cell1/LConn1 -- Solar Cell/LConn1

== system Solar_App/Subsystem4/Subsystem2 ==
  Solar Cell{,1..3} (4 alike) : ee_lib/Sources/Solar Cell  prm=1  Isc=7.34 A  Voc=0.6 V  Is=1e-6 A  Is2=0 A  Iph=7.34 A  Ir0=1000 W/m^2  ec=1.5  N2=2  Rs=0 Ohm  Rp=inf Ohm  N_series=1  TIPH1=0 1/K  EG=1.11 eV  TXIS1=3  TXIS2=3  TRS1=0  TRP1=0  Tmeas=25 degC  TFIXED=25 degC  thermal_mass=100 J/K  initial_temperature=25 degC
      settings: SourceProductBaseCode=PS
  Conn1 : PMIOPort  Side=Left
  Conn2 : PMIOPort  Port=2  Side=Left
  Conn3 : PMIOPort  Port=3  Side=Right
  connections:
  Solar Cell/LConn1 -- Solar Cell1/LConn1 -- Solar Cell2/LConn1 -- Conn1/RConn1 -- Solar Cell3/LConn1
  Conn2/RConn1 -- Solar Cell/LConn2
  Solar Cell1/LConn2 -- Solar Cell/RConn1
  Solar Cell2/LConn2 -- Solar Cell1/RConn1
  Solar Cell3/LConn2 -- Solar Cell2/RConn1
  Conn3/RConn1 -- Solar Cell3/RConn1

== system Solar_App/Subsystem4/Subsystem3 ==
  Solar Cell{,1..3} (4 alike) : ee_lib/Sources/Solar Cell  prm=1  Isc=7.34 A  Voc=0.6 V  Is=1e-6 A  Is2=0 A  Iph=7.34 A  Ir0=1000 W/m^2  ec=1.5  N2=2  Rs=0 Ohm  Rp=inf Ohm  N_series=1  TIPH1=0 1/K  EG=1.11 eV  TXIS1=3  TXIS2=3  TRS1=0  TRP1=0  Tmeas=25 degC  TFIXED=25 degC  thermal_mass=100 J/K  initial_temperature=25 degC
      settings: SourceProductBaseCode=PS
  Conn1 : PMIOPort  Side=Left
  Conn2 : PMIOPort  Port=2  Side=Left
  Conn3 : PMIOPort  Port=3  Side=Right
  connections:
  Conn3/RConn1 -- Solar Cell3/RConn1
  Solar Cell3/LConn2 -- Solar Cell2/RConn1
  Solar Cell2/LConn2 -- Solar Cell1/RConn1
  Solar Cell1/LConn2 -- Solar Cell/RConn1
  Conn2/RConn1 -- Solar Cell/LConn2
  Solar Cell3/LConn1 -- Conn1/RConn1 -- Solar Cell2/LConn1 -- Solar Cell1/LConn1 -- Solar Cell/LConn1

== system Solar_App/Subsystem4/Subsystem4 ==
  Solar Cell{,1..3} (4 alike) : ee_lib/Sources/Solar Cell  prm=1  Isc=7.34 A  Voc=0.6 V  Is=1e-6 A  Is2=0 A  Iph=7.34 A  Ir0=1000 W/m^2  ec=1.5  N2=2  Rs=0 Ohm  Rp=inf Ohm  N_series=1  TIPH1=0 1/K  EG=1.11 eV  TXIS1=3  TXIS2=3  TRS1=0  TRP1=0  Tmeas=25 degC  TFIXED=25 degC  thermal_mass=100 J/K  initial_temperature=25 degC
      settings: SourceProductBaseCode=PS
  Conn1 : PMIOPort  Side=Left
  Conn2 : PMIOPort  Port=2  Side=Left
  Conn3 : PMIOPort  Port=3  Side=Right
  connections:
  Solar Cell/LConn1 -- Solar Cell1/LConn1 -- Solar Cell2/LConn1 -- Conn1/RConn1 -- Solar Cell3/LConn1
  Conn2/RConn1 -- Solar Cell/LConn2
  Solar Cell1/LConn2 -- Solar Cell/RConn1
  Solar Cell2/LConn2 -- Solar Cell1/RConn1
  Solar Cell3/LConn2 -- Solar Cell2/RConn1
  Conn3/RConn1 -- Solar Cell3/RConn1

== system Solar_App/Subsystem5/Subsystem ==
  Solar Cell{,1..3} (4 alike) : ee_lib/Sources/Solar Cell  prm=1  Isc=7.34 A  Voc=0.6 V  Is=1e-6 A  Is2=0 A  Iph=7.34 A  Ir0=1000 W/m^2  ec=1.5  N2=2  Rs=0 Ohm  Rp=inf Ohm  N_series=1  TIPH1=0 1/K  EG=1.11 eV  TXIS1=3  TXIS2=3  TRS1=0  TRP1=0  Tmeas=25 degC  TFIXED=25 degC  thermal_mass=100 J/K  initial_temperature=25 degC
      settings: SourceProductBaseCode=PS
  Conn1 : PMIOPort  Side=Left
  Conn2 : PMIOPort  Port=2  Side=Left
  Conn3 : PMIOPort  Port=3  Side=Right
  connections:
  Conn3/RConn1 -- Solar Cell3/RConn1
  Solar Cell3/LConn2 -- Solar Cell2/RConn1
  Solar Cell2/LConn2 -- Solar Cell1/RConn1
  Solar Cell1/LConn2 -- Solar Cell/RConn1
  Conn2/RConn1 -- Solar Cell/LConn2
  Solar Cell3/LConn1 -- Conn1/RConn1 -- Solar Cell2/LConn1 -- Solar Cell1/LConn1 -- Solar Cell/LConn1

== system Solar_App/Subsystem5/Subsystem1 ==
  Solar Cell{,1..3} (4 alike) : ee_lib/Sources/Solar Cell  prm=1  Isc=7.34 A  Voc=0.6 V  Is=1e-6 A  Is2=0 A  Iph=7.34 A  Ir0=1000 W/m^2  ec=1.5  N2=2  Rs=0 Ohm  Rp=inf Ohm  N_series=1  TIPH1=0 1/K  EG=1.11 eV  TXIS1=3  TXIS2=3  TRS1=0  TRP1=0  Tmeas=25 degC  TFIXED=25 degC  thermal_mass=100 J/K  initial_temperature=25 degC
      settings: SourceProductBaseCode=PS
  Conn1 : PMIOPort  Side=Left
  Conn2 : PMIOPort  Port=2  Side=Left
  Conn3 : PMIOPort  Port=3  Side=Right
  connections:
  Solar Cell/LConn1 -- Solar Cell1/LConn1 -- Solar Cell2/LConn1 -- Conn1/RConn1 -- Solar Cell3/LConn1
  Conn2/RConn1 -- Solar Cell/LConn2
  Solar Cell1/LConn2 -- Solar Cell/RConn1
  Solar Cell2/LConn2 -- Solar Cell1/RConn1
  Solar Cell3/LConn2 -- Solar Cell2/RConn1
  Conn3/RConn1 -- Solar Cell3/RConn1

== system Solar_App/Subsystem5/Subsystem2 ==
  Solar Cell{,1..3} (4 alike) : ee_lib/Sources/Solar Cell  prm=1  Isc=7.34 A  Voc=0.6 V  Is=1e-6 A  Is2=0 A  Iph=7.34 A  Ir0=1000 W/m^2  ec=1.5  N2=2  Rs=0 Ohm  Rp=inf Ohm  N_series=1  TIPH1=0 1/K  EG=1.11 eV  TXIS1=3  TXIS2=3  TRS1=0  TRP1=0  Tmeas=25 degC  TFIXED=25 degC  thermal_mass=100 J/K  initial_temperature=25 degC
      settings: SourceProductBaseCode=PS
  Conn1 : PMIOPort  Side=Left
  Conn2 : PMIOPort  Port=2  Side=Left
  Conn3 : PMIOPort  Port=3  Side=Right
  connections:
  Conn3/RConn1 -- Solar Cell3/RConn1
  Solar Cell3/LConn2 -- Solar Cell2/RConn1
  Solar Cell2/LConn2 -- Solar Cell1/RConn1
  Solar Cell1/LConn2 -- Solar Cell/RConn1
  Conn2/RConn1 -- Solar Cell/LConn2
  Solar Cell3/LConn1 -- Conn1/RConn1 -- Solar Cell2/LConn1 -- Solar Cell1/LConn1 -- Solar Cell/LConn1

== system Solar_App/Subsystem5/Subsystem3 ==
  Solar Cell{,1..3} (4 alike) : ee_lib/Sources/Solar Cell  prm=1  Isc=7.34 A  Voc=0.6 V  Is=1e-6 A  Is2=0 A  Iph=7.34 A  Ir0=1000 W/m^2  ec=1.5  N2=2  Rs=0 Ohm  Rp=inf Ohm  N_series=1  TIPH1=0 1/K  EG=1.11 eV  TXIS1=3  TXIS2=3  TRS1=0  TRP1=0  Tmeas=25 degC  TFIXED=25 degC  thermal_mass=100 J/K  initial_temperature=25 degC
      settings: SourceProductBaseCode=PS
  Conn1 : PMIOPort  Side=Left
  Conn2 : PMIOPort  Port=2  Side=Left
  Conn3 : PMIOPort  Port=3  Side=Right
  connections:
  Solar Cell/LConn1 -- Solar Cell1/LConn1 -- Solar Cell2/LConn1 -- Conn1/RConn1 -- Solar Cell3/LConn1
  Conn2/RConn1 -- Solar Cell/LConn2
  Solar Cell1/LConn2 -- Solar Cell/RConn1
  Solar Cell2/LConn2 -- Solar Cell1/RConn1
  Solar Cell3/LConn2 -- Solar Cell2/RConn1
  Conn3/RConn1 -- Solar Cell3/RConn1

== system Solar_App/Subsystem5/Subsystem4 ==
  Solar Cell{,1..3} (4 alike) : ee_lib/Sources/Solar Cell  prm=1  Isc=7.34 A  Voc=0.6 V  Is=1e-6 A  Is2=0 A  Iph=7.34 A  Ir0=1000 W/m^2  ec=1.5  N2=2  Rs=0 Ohm  Rp=inf Ohm  N_series=1  TIPH1=0 1/K  EG=1.11 eV  TXIS1=3  TXIS2=3  TRS1=0  TRP1=0  Tmeas=25 degC  TFIXED=25 degC  thermal_mass=100 J/K  initial_temperature=25 degC
      settings: SourceProductBaseCode=PS
  Conn1 : PMIOPort  Side=Left
  Conn2 : PMIOPort  Port=2  Side=Left
  Conn3 : PMIOPort  Port=3  Side=Right
  connections:
  Conn3/RConn1 -- Solar Cell3/RConn1
  Solar Cell3/LConn2 -- Solar Cell2/RConn1
  Solar Cell2/LConn2 -- Solar Cell1/RConn1
  Solar Cell1/LConn2 -- Solar Cell/RConn1
  Conn2/RConn1 -- Solar Cell/LConn2
  Solar Cell3/LConn1 -- Conn1/RConn1 -- Solar Cell2/LConn1 -- Solar Cell1/LConn1 -- Solar Cell/LConn1
